simulink model "Copy_of_Quadcopter_Control_PID_Inside_code_and_outside-DESKTOP-UMEUAKD"  (R2021a)
settings: Solver=ode4  StartTime=0.0  StopTime=20  FixedStep=0.01  RelTol=1e-3
settings Model: Creator=Hameed  LastModifiedBy=Hameed

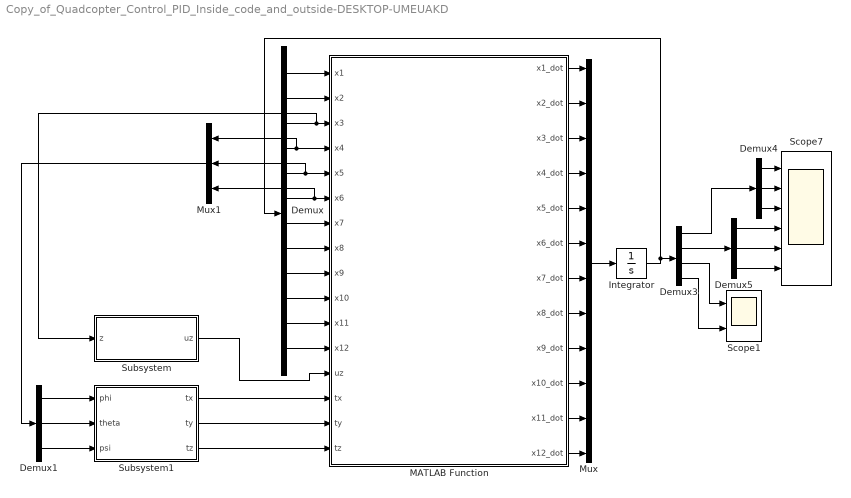
== system Copy_of_Quadcopter_Control_PID_Inside_code_and_outside-DESKTOP-UMEUAKD ==
  Demux : Demux  Outputs=12
  Demux1 : Demux  Outputs=3
  Demux3 : Demux
  Demux4 : Demux  Outputs=3
  Demux5 : Demux  Outputs=3
  Integrator : Integrator  InitialCondition=[0;0;0;0;0;0;0;0;0;0;0;0]
  MATLAB Function : MATLAB Function  TreatAsAtomicUnit=on
  Mux : Mux  Inputs=12
  Mux1 : Mux  Inputs=3
  Scope1 : Scope  NumInputPorts=2
  Scope7 : Scope  NumInputPorts=6
  Subsystem : Subsystem
  Subsystem1 : Subsystem
  wires:
  Subsystem1/3(tz) -> MATLAB Function/16(tz)
  Demux1/1 -> Subsystem1/1(phi)
  MATLAB Function/2(x2_dot) -> Mux/2
  Mux/1 -> Integrator/1
  Demux5/3 -> Scope7/6
  Demux3/3 -> Scope1/1
  Demux4/1 -> Scope7/1
  Mux1/1 -> Demux1/1
  Demux3/4 -> Scope1/2
  Subsystem1/1(tx) -> MATLAB Function/14(tx)
  Demux3/2 -> Demux5/1
  Integrator/1 -> Demux/1, Demux3/1
  Subsystem/1(uz) -> MATLAB Function/13(uz)
  MATLAB Function/1(x1_dot) -> Mux/1
  Demux3/1 -> Demux4/1
  Demux1/2 -> Subsystem1/2(theta)
  MATLAB Function/7(x7_dot) -> Mux/7
  Demux/10 -> MATLAB Function/10(x10)
  MATLAB Function/12(x12_dot) -> Mux/12
  Demux5/2 -> Scope7/5
  MATLAB Function/11(x11_dot) -> Mux/11
  Demux5/1 -> Scope7/4
  MATLAB Function/10(x10_dot) -> Mux/10
  MATLAB Function/4(x4_dot) -> Mux/4
  Demux/11 -> MATLAB Function/11(x11)
  Demux/7 -> MATLAB Function/7(x7)
  Demux/3 -> Subsystem/1(z), MATLAB Function/3(x3)
  Demux/8 -> MATLAB Function/8(x8)
  Demux4/3 -> Scope7/3
  Demux4/2 -> Scope7/2
  MATLAB Function/3(x3_dot) -> Mux/3
  Demux/4 -> MATLAB Function/4(x4), Mux1/1
  MATLAB Function/5(x5_dot) -> Mux/5
  Demux/9 -> MATLAB Function/9(x9)
  Demux/1 -> MATLAB Function/1(x1)
  MATLAB Function/6(x6_dot) -> Mux/6
  Subsystem1/2(ty) -> MATLAB Function/15(ty)
  Demux/2 -> MATLAB Function/2(x2)
  MATLAB Function/9(x9_dot) -> Mux/9
  Demux/12 -> MATLAB Function/12(x12)
  Demux/5 -> Mux1/2, MATLAB Function/5(x5)
  Demux1/3 -> Subsystem1/3(psi)
  Demux/6 -> Mux1/3, MATLAB Function/6(x6)
  MATLAB Function/8(x8_dot) -> Mux/8

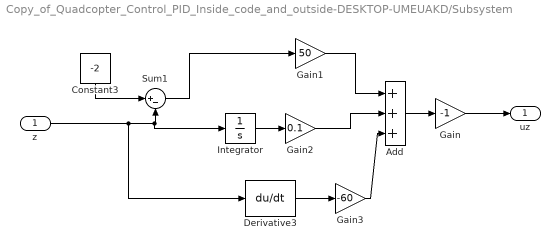
== system Copy_of_Quadcopter_Control_PID_Inside_code_and_outside-DESKTOP-UMEUAKD/Subsystem ==
  z : Inport
  Add : Sum  Inputs=+++
  Constant3 : Constant  Value=-2  VectorParams1D=off
  Derivative3 : Derivative
  Gain : Gain  Gain=-1
  Gain1 : Gain  Gain=50
  Gain2 : Gain  Gain=0.1
  Gain3 : Gain  Gain=-60
  Integrator : Integrator
  Sum1 : Sum  Inputs=|+-
  uz : Outport
  wires:
  Sum1/1 -> Gain1/1
  Add/1 -> Gain/1
  Gain/1 -> uz/1
  z/1 -> Derivative3/1, Integrator/1, Sum1/2
  Constant3/1 -> Sum1/1
  Derivative3/1 -> Gain3/1
  Gain1/1 -> Add/1
  Integrator/1 -> Gain2/1
  Gain2/1 -> Add/2
  Gain3/1 -> Add/3

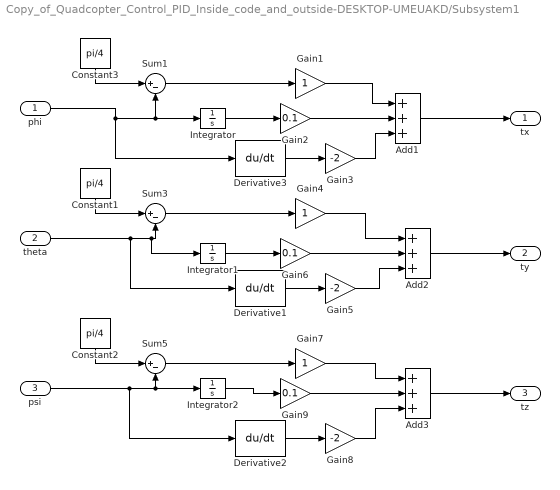
== system Copy_of_Quadcopter_Control_PID_Inside_code_and_outside-DESKTOP-UMEUAKD/Subsystem1 ==
  phi : Inport
  theta : Inport  Port=2
  psi : Inport  Port=3
  Add1 : Sum  Inputs=+++
  Add2 : Sum  Inputs=+++
  Add3 : Sum  Inputs=+++
  Constant1 : Constant  Value=pi/4  VectorParams1D=off
  Constant2 : Constant  Value=pi/4  VectorParams1D=off
  Constant3 : Constant  Value=pi/4  VectorParams1D=off
  Derivative1 : Derivative
  Derivative2 : Derivative
  Derivative3 : Derivative
  Gain1 : Gain
  Gain2 : Gain  Gain=0.1
  Gain3 : Gain  Gain=-2
  Gain4 : Gain
  Gain5 : Gain  Gain=-2
  Gain6 : Gain  Gain=0.1
  Gain7 : Gain
  Gain8 : Gain  Gain=-2
  Gain9 : Gain  Gain=0.1
  Integrator : Integrator
  Integrator1 : Integrator
  Integrator2 : Integrator
  Sum1 : Sum  Inputs=|+-
  Sum3 : Sum  Inputs=|+-
  Sum5 : Sum  Inputs=|+-
  tx : Outport
  ty : Outport  Port=2
  tz : Outport  Port=3
  wires:
  Sum1/1 -> Gain1/1
  Add1/1 -> tx/1
  Constant3/1 -> Sum1/1
  Derivative3/1 -> Gain3/1
  Gain1/1 -> Add1/1
  Gain4/1 -> Add2/1
  Constant1/1 -> Sum3/1
  Sum3/1 -> Gain4/1
  Derivative1/1 -> Gain5/1
  Add3/1 -> tz/1
  Gain7/1 -> Add3/1
  Constant2/1 -> Sum5/1
  Sum5/1 -> Gain7/1
  Derivative2/1 -> Gain8/1
  Integrator/1 -> Gain2/1
  phi/1 -> Sum1/2, Integrator/1, Derivative3/1
  Gain3/1 -> Add1/3
  Gain2/1 -> Add1/2
  theta/1 -> Derivative1/1, Integrator1/1, Sum3/2
  Integrator1/1 -> Gain6/1
  Gain5/1 -> Add2/3
  Gain6/1 -> Add2/2
  Gain8/1 -> Add3/3
  psi/1 -> Derivative2/1, Integrator2/1, Sum5/2
  Integrator2/1 -> Gain9/1
  Gain9/1 -> Add3/2
  Add2/1 -> ty/1

== matlab function Copy_of_Quadcopter_Control_PID_Inside_code_and_outside-DESKTOP-UMEUAKD/MATLAB Function ==
  data: x1 input; x1_dot output; x2 input; x3 input; x4 input; x5 input; x6 input; x7 input; x8 input; x9 input; x10 input; x11 input; x12 input; x2_dot output; x3_dot output; x4_dot output; x5_dot output; x6_dot output; x7_dot output; x8_dot output; x9_dot output; x10_dot output; x11_dot output; x12_dot output; uz input; tx input; ty input; tz input
function [x1_dot,x2_dot,x3_dot,x4_dot,x5_dot,x6_dot,x7_dot,x8_dot,x9_dot,x10_dot,x11_dot,x12_dot]= fcn(x1,x2,x3,x4,x5,x6,x7,x8,x9,x10,x11,x12,uz,tx,ty,tz)

% Ixx= 1.2; 
% Iyy= 1.2;
% Izz= 0.3;
%Izz= 2.3;
%k=1;
k = 1e-3;
L= 0.25;
m= 2;
%km= 0.2;
%km = 0.5e-4;
g= 9.81;
%gamma = km/k; 

Ixx = (1/12)*m*(0.2^2+0.2^2);
Iyy= (1/12)*m*(0.2^2+0.2^2);
Izz= (1/12)*m*(0.2^2+0.2^2);
I= [Ixx 0 0;0 Iyy 0;0 0 Izz];


%R-ZYX Euler
R = [cos(x5)*cos(x6), sin(x4)*sin(x5)*cos(x6)-cos(x4)*sin(x6), cos(x4)*sin(x5)*cos(x6)+sin(x4)*sin(x6);
     cos(x5)*sin(x6), sin(x4)*sin(x5)*sin(x6)+cos(x4)*cos(x6), cos(x4)*sin(x5)*sin(x6)-sin(x4)*cos(x6);
     -sin(x5), sin(x4)*cos(x5), cos(x4)*cos(x5)];


Q = [1 0 -sin(x5);
     0 cos(x4) cos(x5)*sin(x4);
     0 -sin(x4) cos(x5)*cos(x4)];

dQ = [0 0 -cos(x5);
      0 -sin(x4) -sin(x5)*sin(x4)+cos(x5)*cos(x4);
      0 -cos(x4) -sin(x5)*cos(x4)-cos(x5)*sin(x4)];

%P=Q';
%  P=[1 0 0; 
%     0 cos(x4) -sin(x4); 
%     -sin(x5) cos(x5)*sin(x4) cos(x5)*cos(x4)];
%  
 
 
 
M = Q'.*I*Q;

ndot=[x10;x11;x12];

s = Q*ndot;
S = [0 -s(3) s(2);s(3) 0 -s(1);-s(2) s(1) 0];
C = Q'.*S*I*Q + Q'.*I*dQ;

%%-------------------------------------------------------------------

%%---------------------------------------------------

% A = [ 1 1 1 1;
%       0  L 0 -L;
%      -L 0  L  0;
%      gamma -gamma gamma -gamma];
 
%  A = [ 0 0 0 0;
%       0 0 0 0;
%       1 1 1 1;
%       0  L 0 -L;
%      -L 0  L  0;
%      gamma -gamma gamma -gamma];

% 
% %references
% xd = 0; yd = 0; zd = -2;
% phid = pi/4.; thetad = pi/4.; psid = pi/4.;
% 
% %error signals
% ez = zd-x3;
% ephi = phid-x4;
% etheta = thetad-x5;
% epsi = psid-x6;
% 
% %controller
% 
% uz = -(50*ez-60*x9);
% tx = (1*ephi-2*x10);
% ty = (1*etheta-2*x11);
% tz = (1*epsi-2*x12);


%  u = [uz;tx;ty;tz];
%  %u = [0;0;uz;tx;ty;tz];
%  th = pinv(A)*u;
%  w = (th/k);         % actually it's omeega square
% %w= sqrt(th/k);
% % %u=k*A*ws;


 T = uz;
 tB = [tx;ty;tz];

%T = k*(w(1)+w(2)+w(3)+w(4));
%T = k*(w(1)^2+w(2)^2+w(3)^2+w(4)^2);

%tB= [L*k*(w(2)-w(4));L*k*(-w(1)+w(3));km*(w(1)-w(2)+w(3)-w(4))];
%tB= [L*k*(w(2)^2-w(4)^2);L*k*(-w(1)^2+w(3)^2);km*(w(1)^2-w(2)^2+w(3)^2-w(4)^2)];


%Jinv=inv(J)
%x789= g*[0;0;1]-R*[0;0;T]/m;


x789 = (1/m)*(-R*[0;0;T]+ m*g*[0;0;1]);
%x789 = (1/m)*(-k*R*A(1:3,:)*w+ m*g*[0;0;1] );


x101112 = pinv(M)*(tB-C*ndot);
%x101112 = pinv(M)*(Q'*tB-C*ndot);
%x101112= inv(M)*(Q'*k*A(4:6,:)*w -C*ndot );

x1_dot=x7;
x2_dot=x8;
x3_dot=x9;

x4_dot=x10;
x5_dot=x11;
x6_dot=x12;

x7_dot=x789(1);
x8_dot=x789(2);
x9_dot=x789(3);

x10_dot=x101112(1);
x11_dot=x101112(2);
x12_dot=x101112(3);


%%-----------------------------------------------------------------------------













%%-------------------------------------------------------------------------------


% C11=0;
% C12=(Iyy-Izz)*(x11*cos(x4)*sin(x4)+x12*sin(x4)^2*cos(x5))+(Izz-Iyy)*x12*cos(x4)^2*cos(x5)-Ixx*x12*cos(x5);
% C13=(Izz-Iyy)*(x12*cos(x4)*sin(x4)*cos(x5)^2);
% C21=(Izz-Iyy)*(x11*cos(x4)*sin(x4)+x12*sin(x4)*cos(x5))+(Iyy-Izz)*x12*cos(x4)^2*cos(x5)+Ixx*x12*cos(x5);
% C22=(Izz-Iyy)*x10*cos(x4)*sin(x4);
% C23= -Ixx*x12*sin(x5)*cos(x5)+Iyy*x12*sin(x4)^2*sin(x5)*cos(x5)+ Izz*x12*cos(x4)^2*sin(x5)*cos(x5);
% C31=(Iyy-Izz)*(x12*cos(x5)^2*sin(x4)*cos(x4))-Ixx*x11*cos(x5);
% C32= (Izz-Iyy)*(x11*cos(x4)*sin(x4)*sin(x5)+x10*sin(x4)^2*cos(x5))+(Iyy-Izz)*x10*cos(x4)^2*cos(x5)+Ixx*x12*sin(x5)*cos(x5)-Iyy*x12*sin(x10)^2*sin(x5)*cos(x5)-Izz*x12*cos(x10)^2*sin(x5)*cos(x5);
% C33=(Iyy-Izz)*x10*cos(x4)*sin(x4)*cos(x5)^2-Iyy*x11*sin(x4)^2*cos(x5)*sin(x5)-Izz*x11*cos(x4)^2*cos(x5)*sin(x5)+Ixx*x11*cos(x5)*sin(x5);
% C=[C11 C12 C13;C21 C22 C23;C31 C32 C33];
